simulink model "ale_speed_controller"  (R2022a)
settings: configuration reference "ale_config" (kept outside this file)
undefined symbols (not defined in the file or in its folder): framePeriod_s
libraries: slpidlib x2, dspfdesign x1
settings Model: Creator=remoteuser  LastModifiedBy=remoteuser
settings ConfigSetRef: SourceName=ale_config  SourceLocation=Base Workspace

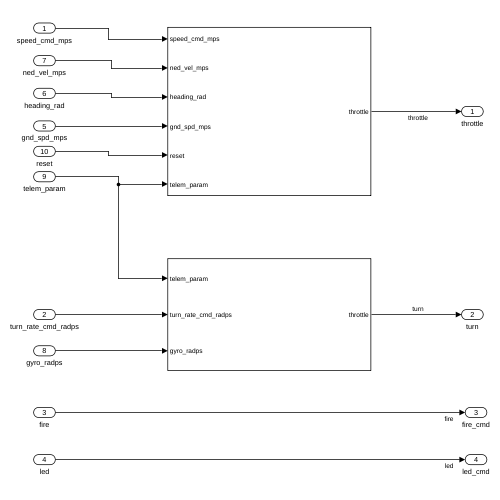
[thumbnail: Simulink's stored preview of the top-level diagram]
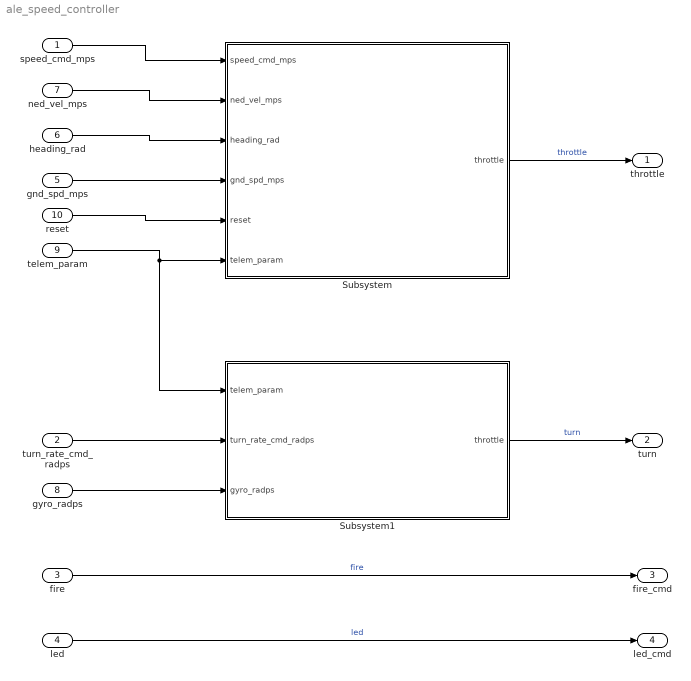
== system ale_speed_controller ==
  speed_cmd_mps : Inport
  turn_rate_cmd_radps : Inport  Port=2
  fire : Inport  Port=3  OutDataTypeStr=single
  led : Inport  Port=4  OutDataTypeStr=single
  gnd_spd_mps : Inport  Port=5  OutDataTypeStr=single
  heading_rad : Inport  Port=6  OutDataTypeStr=single
  ned_vel_mps : Inport  Port=7  OutDataTypeStr=single  PortDimensions=3
  gyro_radps : Inport  Port=8  OutDataTypeStr=single
  telem_param : Inport  Port=9
  reset : Inport  Port=10  OutDataTypeStr=boolean
  Subsystem : Subsystem
  Subsystem1 : Subsystem
  throttle : Outport
  turn : Outport  Port=2
  fire_cmd : Outport  Port=3
  led_cmd : Outport  Port=4
  wires:
  Subsystem1/1(throttle) -> turn/1  "turn"
  fire/1 -> fire_cmd/1  "fire"
  speed_cmd_mps/1 -> Subsystem/1(speed_cmd_mps)
  turn_rate_cmd_radps/1 -> Subsystem1/2(turn_rate_cmd_radps)
  Subsystem/1(throttle) -> throttle/1  "throttle"
  led/1 -> led_cmd/1  "led"
  ned_vel_mps/1 -> Subsystem/2(ned_vel_mps)
  heading_rad/1 -> Subsystem/3(heading_rad)
  gnd_spd_mps/1 -> Subsystem/4(gnd_spd_mps)
  telem_param/1 -> Subsystem1/1(telem_param), Subsystem/6(telem_param)
  gyro_radps/1 -> Subsystem1/3(gyro_radps)
  reset/1 -> Subsystem/5(reset)

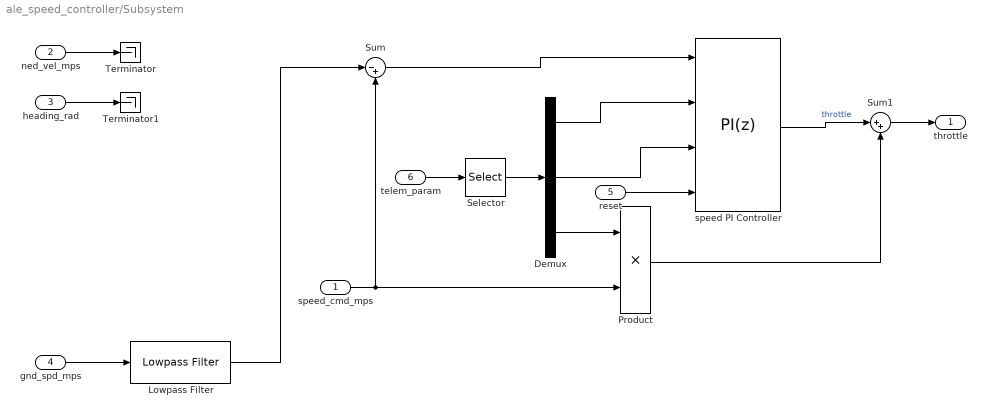
== system ale_speed_controller/Subsystem ==
  speed_cmd_mps : Inport
  ned_vel_mps : Inport  Port=2
  heading_rad : Inport  Port=3
  gnd_spd_mps : Inport  Port=4
  reset : Inport  Port=5
  telem_param : Inport  Port=6
  Demux : Demux  Outputs=3
  Lowpass Filter : dspfdesign/Lowpass Filter  FilterType=FIR  DesignForMinimumOrder=on  FilterOrder=50  PassbandFrequency=2  StopbandFrequency=5  PassbandRipple=0.1  StopbandAttenuation=10  InheritSampleRate=off  SampleRate=50  SimulateUsing=Code generation  roundingMode=Floor  coeffsDataTypeStr=fixdt(1,16)
  Product : Product
  Selector : Selector  IndexMode=Zero-based  IndexOptions=Index vector (dialog)  Indices=[0 1 2]  OutputSizes=1
  Sum : Sum  Inputs=|-+
  Sum1 : Sum  Inputs=|++
  Terminator : Terminator
  Terminator1 : Terminator
  speed PI Controller : slpidlib/PID Controller  Controller=PI  Form=Parallel  TimeDomain=Discrete-time  UseExternalTs=off  SampleTime=framePeriod_s  IntegratorMethod=Forward Euler  FilterMethod=Forward Euler  ControllerParametersSource=external  P=1  I=1  UseKiTs=off  D=0  N=100  UseFilter=on  TunerSelectOption=Transfer Function Based (PID Tuner App)  InitialConditionSource=internal  InitialConditionForIntegrator=0  InitialConditionForFilter=0  DifferentiatorICPrevScaledInput=0  ExternalReset=either  TrackingMode=off  Kt=1  LimitOutput=on  SatLimitsSource=internal  UpperSaturationLimit=1  LowerSaturationLimit=0  LinearizeAsGain=on  AntiWindupMode=clamping  Kb=1  POutMin=[]  POutMax=[]  IOutMin=[]  IOutMax=[]  DOutMin=[]  DOutMax=[]  NOutMin=[]  NOutMax=[]  SumOutMin=[]  SumOutMax=[]  SaturationOutMin=[]  SaturationOutMax=[]  PParamMin=[]  PParamMax=[]  IParamMin=[]  IParamMax=[]  DParamMin=[]  DParamMax=[]  NParamMin=[]  NParamMax=[]  KbParamMin=[]  KbParamMax=[]  KtParamMin=[]  KtParamMax=[]  KbOutMin=[]  KbOutMax=[]  KtOutMin=[]  KtOutMax=[]  IntegratorOutMin=[]  IntegratorOutMax=[]  FilterOutMin=[]  FilterOutMax=[]  SumI1OutMin=[]  SumI1OutMax=[]  SumI2OutMin=[]  SumI2OutMax=[]  SumI3OutMin=[]  SumI3OutMax=[]  SumI4OutMin=[]  SumI4OutMax=[]  SumDOutMin=[]  SumDOutMax=[]  DifferentiatorOutMin=[]  DifferentiatorOutMax=[]  FilterDiffOutCoefMin=[]  FilterDiffOutCoefMax=[]  ReciprocalOutMin=[]  ReciprocalOutMax=[]  SumDenOutMin=[]  SumDenOutMax=[]  SumNumOutMin=[]  SumNumOutMax=[]  DivideOutMin=[]  DivideOutMax=[]  UdiffTsProdOutMin=[]  UdiffTsProdOutMax=[]  NTsProdOutMin=[]  NTsProdOutMax=[]  UintegralTsProdOutMin=[]  UintegralTsProdOutMax=[]  UngainTsProdOutMin=[]  UngainTsProdOutMax=[]  IntegratorContinuousStateAttributes=''  IntegratorStateMustResolveToSignalObject=off  IntegratorRTWStateStorageClass=Auto  FilterContinuousStateAttributes=''  FilterStateMustResolveToSignalObject=off  FilterRTWStateStorageClass=Auto  ParallelPVariant=ExternalParameters  IdealPVariant=Disabled  IVariant=ExternalParameters  DVariant=Disabled  IntegratorVariant=Discrete  SatVariant=Enabled  AWVariant=DiscClampingParallel  PCopyVariant=Disabled  TRVariant=Disabled  FdbkBlocksVariant=Forward  IdealPFdbkVariant=Disabled  SatFdbkVariant=Disabled  DerivativeFilterVariant=Disabled  NVariant=Disabled  NCopyVariant=Disabled_SignalSpec  FilterICVariant=Disabled  IntegratorICVariant=InternalICs  ExternalResetVariant=ExternalReset  TRSumVariant=Passthrough  SumFdbkVariant=Disabled  SumVariant=Sum_PI  TsampFilterVariant=InternalTs  TsampNgainVariant=Passthrough  TsampIntegralVariant=Passthrough  ExternalSaturationOutDataTypeStr=Inherit: Same as second input  aMode=0
  throttle : Outport
  wires:
  Product/1 -> Sum1/2
  Demux/3 -> Product/1
  Sum1/1 -> throttle/1
  speed PI Controller/1 -> Sum1/1  "throttle"
  gnd_spd_mps/1 -> Lowpass Filter/1
  Lowpass Filter/1 -> Sum/1
  speed_cmd_mps/1 -> Product/2, Sum/2
  heading_rad/1 -> Terminator1/1
  ned_vel_mps/1 -> Terminator/1
  Selector/1 -> Demux/1
  Demux/2 -> speed PI Controller/3
  Demux/1 -> speed PI Controller/2
  telem_param/1 -> Selector/1
  Sum/1 -> speed PI Controller/1
  reset/1 -> speed PI Controller/4

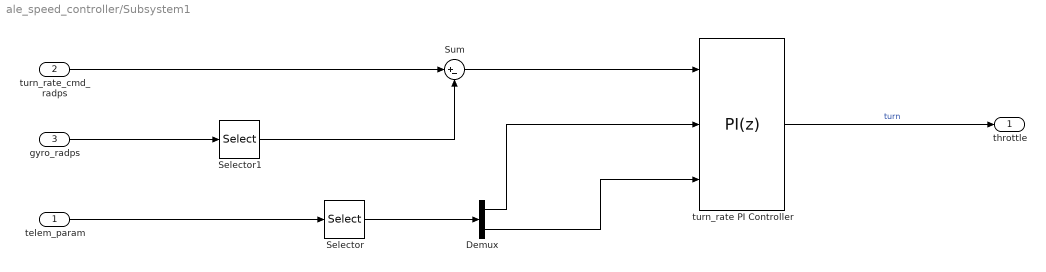
== system ale_speed_controller/Subsystem1 ==
  telem_param : Inport
  turn_rate_cmd_radps : Inport  Port=2
  gyro_radps : Inport  Port=3
  Demux : Demux  Outputs=2
  Selector : Selector  IndexMode=Zero-based  InputPortWidth=24  IndexOptions=Index vector (dialog)  Indices=[3 4]  OutputSizes=1
  Selector1 : Selector  InputPortWidth=3  IndexOptions=Index vector (dialog)  Indices=3  OutputSizes=1
  Sum : Sum  Inputs=|+-
  turn_rate PI Controller : slpidlib/PID Controller  Controller=PI  Form=Parallel  TimeDomain=Discrete-time  UseExternalTs=off  SampleTime=framePeriod_s  IntegratorMethod=Forward Euler  FilterMethod=Forward Euler  ControllerParametersSource=external  P=1  I=1  UseKiTs=off  D=0  N=100  UseFilter=on  TunerSelectOption=Transfer Function Based (PID Tuner App)  InitialConditionSource=internal  InitialConditionForIntegrator=0  InitialConditionForFilter=0  DifferentiatorICPrevScaledInput=0  ExternalReset=none  TrackingMode=off  Kt=1  LimitOutput=on  SatLimitsSource=internal  UpperSaturationLimit=1  LowerSaturationLimit=-1  LinearizeAsGain=on  AntiWindupMode=clamping  Kb=1  POutMin=[]  POutMax=[]  IOutMin=[]  IOutMax=[]  DOutMin=[]  DOutMax=[]  NOutMin=[]  NOutMax=[]  SumOutMin=[]  SumOutMax=[]  SaturationOutMin=[]  SaturationOutMax=[]  PParamMin=[]  PParamMax=[]  IParamMin=[]  IParamMax=[]  DParamMin=[]  DParamMax=[]  NParamMin=[]  NParamMax=[]  KbParamMin=[]  KbParamMax=[]  KtParamMin=[]  KtParamMax=[]  KbOutMin=[]  KbOutMax=[]  KtOutMin=[]  KtOutMax=[]  IntegratorOutMin=[]  IntegratorOutMax=[]  FilterOutMin=[]  FilterOutMax=[]  SumI1OutMin=[]  SumI1OutMax=[]  SumI2OutMin=[]  SumI2OutMax=[]  SumI3OutMin=[]  SumI3OutMax=[]  SumI4OutMin=[]  SumI4OutMax=[]  SumDOutMin=[]  SumDOutMax=[]  DifferentiatorOutMin=[]  DifferentiatorOutMax=[]  FilterDiffOutCoefMin=[]  FilterDiffOutCoefMax=[]  ReciprocalOutMin=[]  ReciprocalOutMax=[]  SumDenOutMin=[]  SumDenOutMax=[]  SumNumOutMin=[]  SumNumOutMax=[]  DivideOutMin=[]  DivideOutMax=[]  UdiffTsProdOutMin=[]  UdiffTsProdOutMax=[]  NTsProdOutMin=[]  NTsProdOutMax=[]  UintegralTsProdOutMin=[]  UintegralTsProdOutMax=[]  UngainTsProdOutMin=[]  UngainTsProdOutMax=[]  IntegratorContinuousStateAttributes=''  IntegratorStateMustResolveToSignalObject=off  IntegratorRTWStateStorageClass=Auto  FilterContinuousStateAttributes=''  FilterStateMustResolveToSignalObject=off  FilterRTWStateStorageClass=Auto  ParallelPVariant=ExternalParameters  IdealPVariant=Disabled  IVariant=ExternalParameters  DVariant=Disabled  IntegratorVariant=Discrete  SatVariant=Enabled  AWVariant=DiscClampingParallel  PCopyVariant=Disabled  TRVariant=Disabled  FdbkBlocksVariant=Forward  IdealPFdbkVariant=Disabled  SatFdbkVariant=Disabled  DerivativeFilterVariant=Disabled  NVariant=Disabled  NCopyVariant=Disabled_SignalSpec  FilterICVariant=Disabled  IntegratorICVariant=InternalICs  ExternalResetVariant=Disabled  TRSumVariant=Passthrough  SumFdbkVariant=Disabled  SumVariant=Sum_PI  TsampFilterVariant=InternalTs  TsampNgainVariant=Passthrough  TsampIntegralVariant=Passthrough  ExternalSaturationOutDataTypeStr=Inherit: Same as second input  aMode=0
  throttle : Outport
  wires:
  Demux/2 -> turn_rate PI Controller/3
  Demux/1 -> turn_rate PI Controller/2
  Selector/1 -> Demux/1
  gyro_radps/1 -> Selector1/1
  turn_rate PI Controller/1 -> throttle/1  "turn"
  Sum/1 -> turn_rate PI Controller/1
  Selector1/1 -> Sum/2
  turn_rate_cmd_radps/1 -> Sum/1
  telem_param/1 -> Selector/1
